simulink model "ARC_DTm"  (R2025b)
settings: Solver=FixedStepAuto  StartTime=0.0  StopTime=10080  FixedStep=1  RelTol=1e-3
PreLoadFcn:
  | %For Preload, set the working path
  | modelFolder = fileparts(which(bdroot));
  | addpath(genpath(modelFolder));
StartFcn:
  | tic
StopFcn:
  | fprintf("Sim Time: %.02f min", toc/60)
values from neighbouring files (symbols this model uses):
  batteryScenario = p.batteryScenario    [RUNSIM_ParameterSweep.m]    (also in _RUNSIM_ParameterSweep.m)
  Electricity_SalePriceModifier = 50/100    (= 0.5)    [RUNSIM_ParameterSweep.m]    (also in _RUNSIM_ParameterSweep.m)
  LUT = LUT_load.gamLUT    [RUNSIM_ParameterSweep.m]    (also in _RUNSIM_ParameterSweep.m)
  minimum_UF_system_flow = 5833    [RUNSIM_ParameterSweep.m]    (also in _RUNSIM_ParameterSweep.m)
  PROS1_recoveryrate = 61    [RUNSIM_ParameterSweep.m]    (also in _RUNSIM_ParameterSweep.m)
  PROS2_recoveryrate = 62    [RUNSIM_ParameterSweep.m]    (also in _RUNSIM_ParameterSweep.m)
  ROstabilization_time = p.ROstabilization_time    [RUNSIM_ParameterSweep.m]    (also in _RUNSIM_ParameterSweep.m)
  solarModifier = maximum_solar_generation / 300    [RUNSIM_ParameterSweep.m]    (also in _RUNSIM_ParameterSweep.m)
  TSRO_recoveryrate = 51    [RUNSIM_ParameterSweep.m]    (also in _RUNSIM_ParameterSweep.m)
  UF_RecoveryRate = 96    [RUNSIM_ParameterSweep.m]    (also in _RUNSIM_ParameterSweep.m)
undefined symbols (not defined in the file or in its folder): A_PROS1, A_PROS2, A_TSRO, B_PROS1, B_PROS2, B_TSRO, BW_Max_Time, BW_Max_Vol_gal, CEB_Max_Time, CEB_Max_Vol_gal, CIP_Max_Time, E, FF, h, L, w
libraries: simulink x40
(part 5 of 11)

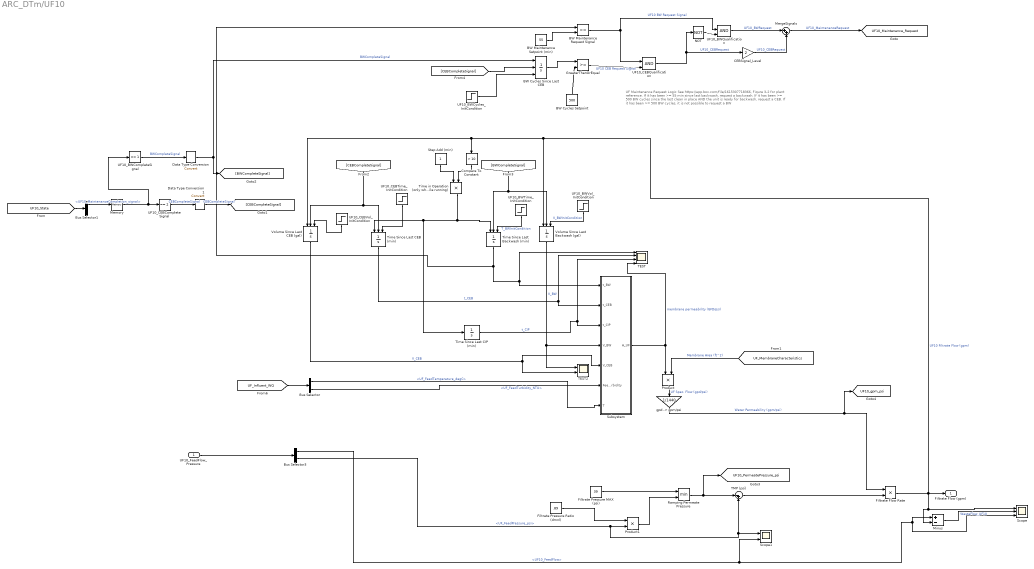
== system ARC_DTm/UF10 ==
  note: UF Maintenance Request Logic
      | See https://app.box.com/file/1615307718366, Figure 3-2 for plant reference.
      |
      | If it has been >= 55 min since last backwash, request a backwash.
      | If it has been >= 500 BW cycles since the last clean in place AND the unit is ready for backwash, request a CEB.
      | If it has been >= 500 BW cycles, it is not possible to request a BW
  UF10_FeedFlow_Pressure : Inport
  BW Cycles Setpoint : Constant  Value=500
  BW Cycles Since Last CEB : Integrator  ExternalReset=rising  InitialConditionSource=external  InitialCondition=5
  BW Maintenance Request Signal : RelationalOperator  OutDataTypeStr=boolean  RndMeth=Simplest  InputSameDT=off
  BW Maintenance Setpoint (min) : Constant  Value=55
  Bus Selector : BusSelector  OutputSignals=UF_FeedTemperature_degC,UF_FeedTurbidity_NTU
  Bus Selector1 : BusSelector  OutputSignals=UF10_MaintenanceCompletion_signal,UF10_OperationsState_signal
  Bus Selector3 : BusSelector  OutputSignals=UF10_FeedFlow,UF_FeedPressure_psi
  CEBSignal_Level : Gain  Gain=2  OutDataTypeStr=double
  Compare To Constant : simulink/Logic and Bit Operations/Compare To Constant  relop=>  const=10  OutDataTypeStr=boolean
  Data Type Conversion : DataTypeConversion  SaturateOnIntegerOverflow=off  RndMeth=Floor
  Data Type Conversion1 : DataTypeConversion  SaturateOnIntegerOverflow=off  RndMeth=Floor
  Filtrate Flow Rate : Product
  Filtrate Pressure MAX (psi) : Constant  Value=39
  Filtrate Pressure Ratio (dmnl) : Constant  Value=.89
  GreaterThanOrEqual : RelationalOperator  OutDataTypeStr=boolean  RndMeth=Simplest  InputSameDT=off
  Memory : Memory
  MergeSignals : Sum  Inputs=|++
  Minus : Sum  Inputs=+-
  NOT : Logic  Operator=NOT  IconShape=distinctive  AllPortsSameDT=off  OutDataTypeStr=boolean
  Product : Product
  Product1 : Product
  Ramping Permeate Pressure : MinMax  Inputs=2
  Scope : Scope  NumInputPorts=3
      settings: ActiveDisplayYMinimum=-126.71796384165732  ActiveDisplayYMaximum=1140.4616745749161  DataLoggingVariableName=ScopeData10
  Scope1 : Scope  NumInputPorts=2
      settings: ActiveDisplayYMinimum=-129.2228584451866  ActiveDisplayYMaximum=1163.0057260066797  DataLoggingVariableName=ScopeData11
  Step Add (min) : Constant
  Subsystem : Subsystem
  TEST : Scope  NumInputPorts=4
      settings: ActiveDisplayYMinimum=13.625  ActiveDisplayYMaximum=27.375  DataLoggingVariableName=ScopeData3
  TEST2 : Scope  NumInputPorts=2
      settings: ActiveDisplayYMinimum=-311929.86683332996  ActiveDisplayYMaximum=2.8073688014999703E+6  DataLoggingVariableName=ScopeData4
  TMP (psi) : Sum  Inputs=|-+
  Time Since Last Backwash (min) : Integrator  ExternalReset=level hold  InitialConditionSource=external  InitialCondition=26
  Time Since Last CEB (min) : Integrator  ExternalReset=level hold  InitialConditionSource=external  InitialCondition=4833
  Time Since Last CIP (min) : Integrator  InitialCondition=round(CIP_Max_Time*rand())
  Time in Operation (only while running) : Product
  UF10_BWCompleteSignal : simulink/Logic and Bit Operations/Compare To Constant  relop===  const=1  OutDataTypeStr=uint8
  UF10_BWCycles_InitCondition : Step  Before=round(500 * rand())  After=0  SampleTime=0
  UF10_BWQualification : Logic  IconShape=distinctive  AllPortsSameDT=off  OutDataTypeStr=boolean
  UF10_BWTime_InitCondition : Step  Before=round(BW_Max_Time*rand())  After=0  SampleTime=0
  UF10_BWVol_InitCondition : Step  Before=round(BW_Max_Vol_gal*rand())  After=0  SampleTime=0
  UF10_CEBCompleteSignal : simulink/Logic and Bit Operations/Compare To Constant  relop===  const=2  OutDataTypeStr=uint8
  UF10_CEBQualification : Logic  IconShape=distinctive  AllPortsSameDT=off  OutDataTypeStr=boolean
  UF10_CEBTime_InitCondition : Step  Before=round(CEB_Max_Time*rand())  After=0  SampleTime=0
  UF10_CEBVol_InitCondition : Step  Before=round(CEB_Max_Vol_gal*rand())  After=0  SampleTime=0
  Volume Since Last Backwash (gal) : Integrator  ExternalReset=level hold  InitialConditionSource=external  InitialCondition=34330
  Volume Since Last CEB (gal) : Integrator  ExternalReset=rising  InitialConditionSource=external  InitialCondition=2777254
  "gpd -> gpm/psi" : Gain  Gain=1/1440
  Filtrate Flow (gpm) : Outport
  tag scope: UF10_Maintenance_Request=global, UF10_PermeatePressure_psi=global, UF10_gpm_psi=global
  wires:
  Volume Since Last Backwash (gal)/1 -> Subsystem/4(V_BW), TEST2/1  "V_BW"
  Time Since Last Backwash (min)/1 -> BW Maintenance Request Signal/1, Subsystem/1(t_BW), TEST/1
  Product/1 -> "gpd -> gpm/psi"/1  "UF Spec. Flow (gpd/psi)"
  [UF_MembraneCharacteristics] -> Product/2  "Membrane Area (ft^2)"
  "gpd -> gpm/psi"/1 -> Filtrate Flow Rate/1, [UF10_gpm_psi]  "Water Permeability (gpm/psi)"
  Time in Operation (only while running)/1 -> Time Since Last Backwash (min)/1, Time Since Last CEB (min)/1, Time Since Last CIP (min)/1
  Filtrate Flow Rate/1 -> Scope/1, Minus/2, Volume Since Last Backwash (gal)/1, Volume Since Last CEB (gal)/1, Compare To Constant/1, Filtrate Flow (gpm)/1  "UF10 Filtrate Flow (gpm)"
  Time Since Last CEB (min)/1 -> Subsystem/2(t_CEB), TEST/2  "t_CEB"
  Volume Since Last CEB (gal)/1 -> Subsystem/5(V_CEB), TEST2/2  "V_CEB"
  Time Since Last CIP (min)/1 -> Subsystem/3(t_CIP), TEST/3  "t_CIP"
  Filtrate Pressure MAX (psi)/1 -> Ramping Permeate Pressure/1
  [UF_Influent_WQ] -> Bus Selector/1
  Bus Selector/1 -> Subsystem/7(T)  "<UF_FeedTemperature_degC>"
  UF10_FeedFlow_Pressure/1 -> Bus Selector3/1
  Filtrate Pressure Ratio (dmnl)/1 -> Product1/1
  Product1/1 -> Ramping Permeate Pressure/2
  Ramping Permeate Pressure/1 -> [UF10_PermeatePressure_psi], TMP (psi)/1
  TMP (psi)/1 -> Filtrate Flow Rate/2
  BW Maintenance Setpoint (min)/1 -> BW Maintenance Request Signal/2
  BW Cycles Since Last CEB/1 -> GreaterThanOrEqual/1
  BW Cycles Setpoint/1 -> GreaterThanOrEqual/2
  Bus Selector/2 -> Subsystem/6(Feed Turbidity)  "<UF_FeedTurbidity_NTU>"
  [UF10_State] -> Bus Selector1/1
  MergeSignals/1 -> [UF10_Maintenance_Request]  "UF10_MaintenanceRequest"
  UF10_CEBCompleteSignal/1 -> Data Type Conversion1/1  "CEBCompleteSignal"
  [CEBCompleteSignal] -> Volume Since Last CEB (gal)/2, Time Since Last CEB (min)/2
  Data Type Conversion/1 -> [BWCompleteSignal], BW Cycles Since Last CEB/1  "BWCompleteSignal"
  [BWCompleteSignal] -> Volume Since Last Backwash (gal)/2, Time Since Last Backwash (min)/2
  [CEBCompleteSignal] -> BW Cycles Since Last CEB/2
  Bus Selector1/1 -> Memory/1  "<UF10_MaintenanceCompletion_signal>"
  UF10_BWCompleteSignal/1 -> Data Type Conversion/1  "BWCompleteSignal"
  Data Type Conversion1/1 -> [CEBCompleteSignal]  "CEBCompleteSignal"
  UF10_BWCycles_InitCondition/1 -> BW Cycles Since Last CEB/3
  Subsystem/1(A_UF) -> TEST/4, Product/1  "membrane permeability (GFD/psi)"
  UF10_BWTime_InitCondition/1 -> Time Since Last Backwash (min)/3  "T_BWInitCondition"
  UF10_CEBVol_InitCondition/1 -> Volume Since Last CEB (gal)/3
  UF10_CEBTime_InitCondition/1 -> Time Since Last CEB (min)/3
  UF10_BWVol_InitCondition/1 -> Volume Since Last Backwash (gal)/3  "V_BWInitCondition"
  Step Add (min)/1 -> Time in Operation (only while running)/1
  Compare To Constant/1 -> Time in Operation (only while running)/2
  Memory/1 -> UF10_BWCompleteSignal/1, UF10_CEBCompleteSignal/1
  UF10_BWQualification/1 -> MergeSignals/1  "UF10_BWRequest"
  GreaterThanOrEqual/1 -> UF10_CEBQualification/2  "UF10 CEB Request Signal"
  UF10_CEBQualification/1 -> CEBSignal_Level/1, NOT/1  "UF10_CEBRequest"
  BW Maintenance Request Signal/1 -> UF10_BWQualification/1, UF10_CEBQualification/1  "UF10 BW Request Signal"
  NOT/1 -> UF10_BWQualification/2
  CEBSignal_Level/1 -> MergeSignals/2  "UF10_CEBRequest"
  Bus Selector3/1 -> Scope1/2, Minus/1, Scope/3  "<UF10_FeedFlow>"
  Bus Selector3/2 -> TMP (psi)/2, Scope1/1, Product1/2  "<UF_FeedPressure_psi>"
  Minus/1 -> Scope/2  "WasteFlow_UF10"

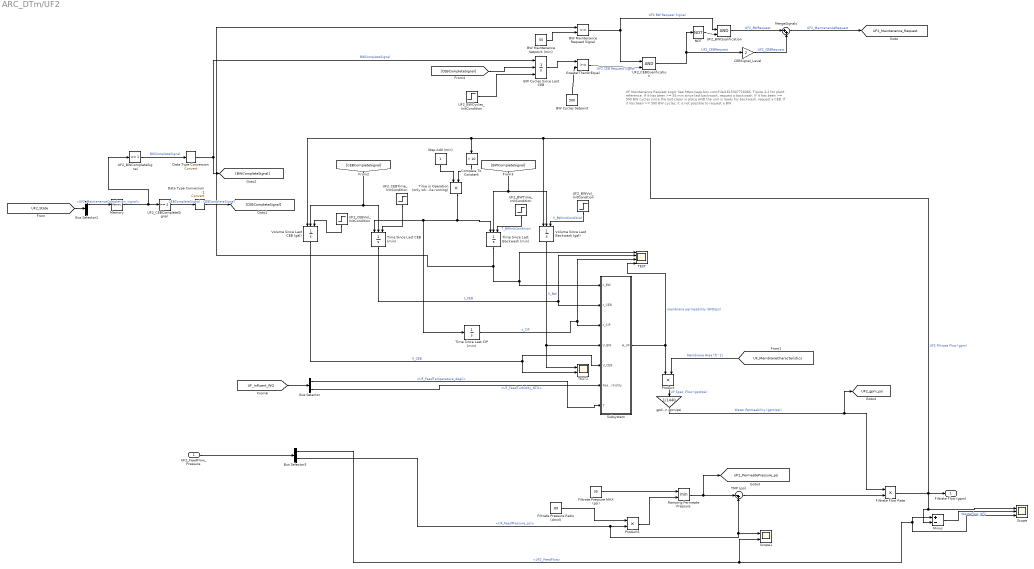
== system ARC_DTm/UF2 ==
  note: UF Maintenance Request Logic
      | See https://app.box.com/file/1615307718366, Figure 3-2 for plant reference.
      |
      | If it has been >= 55 min since last backwash, request a backwash.
      | If it has been >= 500 BW cycles since the last clean in place AND the unit is ready for backwash, request a CEB.
      | If it has been >= 500 BW cycles, it is not possible to request a BW
  UF2_FeedFlow_Pressure : Inport
  BW Cycles Setpoint : Constant  Value=500
  BW Cycles Since Last CEB : Integrator  ExternalReset=rising  InitialConditionSource=external  InitialCondition=5
  BW Maintenance Request Signal : RelationalOperator  OutDataTypeStr=boolean  RndMeth=Simplest  InputSameDT=off
  BW Maintenance Setpoint (min) : Constant  Value=55
  Bus Selector : BusSelector  OutputSignals=UF_FeedTemperature_degC,UF_FeedTurbidity_NTU
  Bus Selector1 : BusSelector  OutputSignals=UF2_MaintenanceCompletion_signal,UF2_OperationsState_signal
  Bus Selector3 : BusSelector  OutputSignals=UF2_FeedFlow,UF_FeedPressure_psi
  CEBSignal_Level : Gain  Gain=2  OutDataTypeStr=double
  Compare To Constant : simulink/Logic and Bit Operations/Compare To Constant  relop=>  const=10  OutDataTypeStr=boolean
  Data Type Conversion : DataTypeConversion  SaturateOnIntegerOverflow=off  RndMeth=Floor
  Data Type Conversion1 : DataTypeConversion  SaturateOnIntegerOverflow=off  RndMeth=Floor
  Filtrate Flow Rate : Product
  Filtrate Pressure MAX (psi) : Constant  Value=39
  Filtrate Pressure Ratio (dmnl) : Constant  Value=.89
  GreaterThanOrEqual : RelationalOperator  OutDataTypeStr=boolean  RndMeth=Simplest  InputSameDT=off
  Memory : Memory
  MergeSignals : Sum  Inputs=|++
  Minus : Sum  Inputs=+-
  NOT : Logic  Operator=NOT  IconShape=distinctive  AllPortsSameDT=off  OutDataTypeStr=boolean
  Product : Product
  Product1 : Product
  Ramping Permeate Pressure : MinMax  Inputs=2
  Scope : Scope  NumInputPorts=3
      settings: ActiveDisplayYMinimum=-126.71796384165732  ActiveDisplayYMaximum=1140.4616745749161  DataLoggingVariableName=ScopeData10
  Scope1 : Scope  NumInputPorts=2
      settings: ActiveDisplayYMinimum=-129.2228584451866  ActiveDisplayYMaximum=1163.0057260066797  DataLoggingVariableName=ScopeData11
  Step Add (min) : Constant
  Subsystem : Subsystem
  TEST : Scope  NumInputPorts=4
      settings: ActiveDisplayYMinimum=13.625  ActiveDisplayYMaximum=27.375  DataLoggingVariableName=ScopeData3
  TEST2 : Scope  NumInputPorts=2
      settings: ActiveDisplayYMinimum=-311929.86683332996  ActiveDisplayYMaximum=2.8073688014999703E+6  DataLoggingVariableName=ScopeData4
  TMP (psi) : Sum  Inputs=|-+
  Time Since Last Backwash (min) : Integrator  ExternalReset=level hold  InitialConditionSource=external  InitialCondition=26
  Time Since Last CEB (min) : Integrator  ExternalReset=level hold  InitialConditionSource=external  InitialCondition=4833
  Time Since Last CIP (min) : Integrator  InitialCondition=round(CIP_Max_Time*rand())
  Time in Operation (only while running) : Product
  UF2_BWCompleteSignal : simulink/Logic and Bit Operations/Compare To Constant  relop===  const=1  OutDataTypeStr=uint8
  UF2_BWCycles_InitCondition : Step  Before=round(500 * rand())  After=0  SampleTime=0
  UF2_BWQualification : Logic  IconShape=distinctive  AllPortsSameDT=off  OutDataTypeStr=boolean
  UF2_BWTime_InitCondition : Step  Before=round(BW_Max_Time*rand())  After=0  SampleTime=0
  UF2_BWVol_InitCondition : Step  Before=round(BW_Max_Vol_gal*rand())  After=0  SampleTime=0
  UF2_CEBCompleteSignal : simulink/Logic and Bit Operations/Compare To Constant  relop===  const=2  OutDataTypeStr=uint8
  UF2_CEBQualification : Logic  IconShape=distinctive  AllPortsSameDT=off  OutDataTypeStr=boolean
  UF2_CEBTime_InitCondition : Step  Before=round(CEB_Max_Time*rand())  After=0  SampleTime=0
  UF2_CEBVol_InitCondition : Step  Before=round(CEB_Max_Vol_gal*rand())  After=0  SampleTime=0
  Volume Since Last Backwash (gal) : Integrator  ExternalReset=level hold  InitialConditionSource=external  InitialCondition=34330
  Volume Since Last CEB (gal) : Integrator  ExternalReset=rising  InitialConditionSource=external  InitialCondition=2777254
  "gpd -> gpm/psi" : Gain  Gain=1/1440
  Filtrate Flow (gpm) : Outport
  tag scope: UF2_Maintenance_Request=global, UF2_PermeatePressure_psi=global, UF2_gpm_psi=global
  wires:
  Volume Since Last Backwash (gal)/1 -> Subsystem/4(V_BW), TEST2/1  "V_BW"
  Time Since Last Backwash (min)/1 -> BW Maintenance Request Signal/1, Subsystem/1(t_BW), TEST/1
  Product/1 -> "gpd -> gpm/psi"/1  "UF Spec. Flow (gpd/psi)"
  [UF_MembraneCharacteristics] -> Product/2  "Membrane Area (ft^2)"
  "gpd -> gpm/psi"/1 -> Filtrate Flow Rate/1, [UF2_gpm_psi]  "Water Permeability (gpm/psi)"
  Time in Operation (only while running)/1 -> Time Since Last Backwash (min)/1, Time Since Last CEB (min)/1, Time Since Last CIP (min)/1
  Filtrate Flow Rate/1 -> Scope/1, Minus/2, Volume Since Last Backwash (gal)/1, Volume Since Last CEB (gal)/1, Compare To Constant/1, Filtrate Flow (gpm)/1  "UF2 Filtrate Flow (gpm)"
  Time Since Last CEB (min)/1 -> Subsystem/2(t_CEB), TEST/2  "t_CEB"
  Volume Since Last CEB (gal)/1 -> Subsystem/5(V_CEB), TEST2/2  "V_CEB"
  Time Since Last CIP (min)/1 -> Subsystem/3(t_CIP), TEST/3  "t_CIP"
  Filtrate Pressure MAX (psi)/1 -> Ramping Permeate Pressure/1
  [UF_Influent_WQ] -> Bus Selector/1
  Bus Selector/1 -> Subsystem/7(T)  "<UF_FeedTemperature_degC>"
  UF2_FeedFlow_Pressure/1 -> Bus Selector3/1
  Filtrate Pressure Ratio (dmnl)/1 -> Product1/1
  Product1/1 -> Ramping Permeate Pressure/2
  Ramping Permeate Pressure/1 -> [UF2_PermeatePressure_psi], TMP (psi)/1
  TMP (psi)/1 -> Filtrate Flow Rate/2
  BW Maintenance Setpoint (min)/1 -> BW Maintenance Request Signal/2
  BW Cycles Since Last CEB/1 -> GreaterThanOrEqual/1
  BW Cycles Setpoint/1 -> GreaterThanOrEqual/2
  Bus Selector/2 -> Subsystem/6(Feed Turbidity)  "<UF_FeedTurbidity_NTU>"
  [UF2_State] -> Bus Selector1/1
  MergeSignals/1 -> [UF2_Maintenance_Request]  "UF2_MaintenanceRequest"
  UF2_CEBCompleteSignal/1 -> Data Type Conversion1/1  "CEBCompleteSignal"
  [CEBCompleteSignal] -> Volume Since Last CEB (gal)/2, Time Since Last CEB (min)/2
  Data Type Conversion/1 -> [BWCompleteSignal], BW Cycles Since Last CEB/1  "BWCompleteSignal"
  [BWCompleteSignal] -> Volume Since Last Backwash (gal)/2, Time Since Last Backwash (min)/2
  [CEBCompleteSignal] -> BW Cycles Since Last CEB/2
  Bus Selector1/1 -> Memory/1  "<UF2_MaintenanceCompletion_signal>"
  UF2_BWCompleteSignal/1 -> Data Type Conversion/1  "BWCompleteSignal"
  Data Type Conversion1/1 -> [CEBCompleteSignal]  "CEBCompleteSignal"
  UF2_BWCycles_InitCondition/1 -> BW Cycles Since Last CEB/3
  Subsystem/1(A_UF) -> TEST/4, Product/1  "membrane permeability (GFD/psi)"
  UF2_BWTime_InitCondition/1 -> Time Since Last Backwash (min)/3  "T_BWInitCondition"
  UF2_CEBVol_InitCondition/1 -> Volume Since Last CEB (gal)/3
  UF2_CEBTime_InitCondition/1 -> Time Since Last CEB (min)/3
  UF2_BWVol_InitCondition/1 -> Volume Since Last Backwash (gal)/3  "V_BWInitCondition"
  Step Add (min)/1 -> Time in Operation (only while running)/1
  Compare To Constant/1 -> Time in Operation (only while running)/2
  Memory/1 -> UF2_BWCompleteSignal/1, UF2_CEBCompleteSignal/1
  UF2_BWQualification/1 -> MergeSignals/1  "UF2_BWRequest"
  GreaterThanOrEqual/1 -> UF2_CEBQualification/2  "UF2 CEB Request Signal"
  UF2_CEBQualification/1 -> CEBSignal_Level/1, NOT/1  "UF2_CEBRequest"
  BW Maintenance Request Signal/1 -> UF2_BWQualification/1, UF2_CEBQualification/1  "UF2 BW Request Signal"
  NOT/1 -> UF2_BWQualification/2
  CEBSignal_Level/1 -> MergeSignals/2  "UF2_CEBRequest"
  Bus Selector3/1 -> Scope1/2, Minus/1, Scope/3  "<UF2_FeedFlow>"
  Bus Selector3/2 -> TMP (psi)/2, Scope1/1, Product1/2  "<UF_FeedPressure_psi>"
  Minus/1 -> Scope/2  "WasteFlow_UF2"

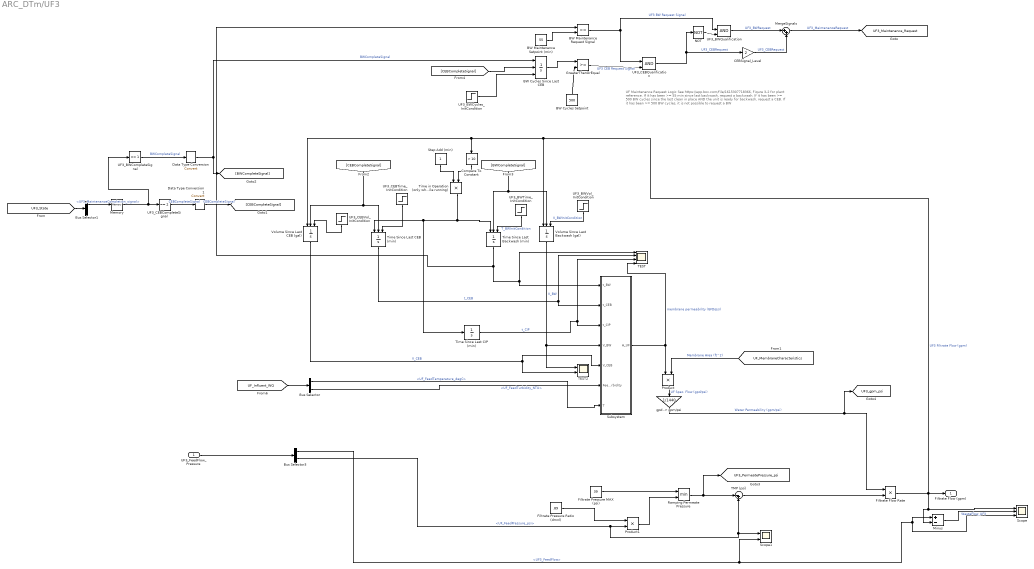
== system ARC_DTm/UF3 ==
  note: UF Maintenance Request Logic
      | See https://app.box.com/file/1615307718366, Figure 3-2 for plant reference.
      |
      | If it has been >= 55 min since last backwash, request a backwash.
      | If it has been >= 500 BW cycles since the last clean in place AND the unit is ready for backwash, request a CEB.
      | If it has been >= 500 BW cycles, it is not possible to request a BW
  UF3_FeedFlow_Pressure : Inport
  BW Cycles Setpoint : Constant  Value=500
  BW Cycles Since Last CEB : Integrator  ExternalReset=rising  InitialConditionSource=external  InitialCondition=5
  BW Maintenance Request Signal : RelationalOperator  OutDataTypeStr=boolean  RndMeth=Simplest  InputSameDT=off
  BW Maintenance Setpoint (min) : Constant  Value=55
  Bus Selector : BusSelector  OutputSignals=UF_FeedTemperature_degC,UF_FeedTurbidity_NTU
  Bus Selector1 : BusSelector  OutputSignals=UF3_MaintenanceCompletion_signal,UF3_OperationsState_signal
  Bus Selector3 : BusSelector  OutputSignals=UF3_FeedFlow,UF_FeedPressure_psi
  CEBSignal_Level : Gain  Gain=2  OutDataTypeStr=double
  Compare To Constant : simulink/Logic and Bit Operations/Compare To Constant  relop=>  const=10  OutDataTypeStr=boolean
  Data Type Conversion : DataTypeConversion  SaturateOnIntegerOverflow=off  RndMeth=Floor
  Data Type Conversion1 : DataTypeConversion  SaturateOnIntegerOverflow=off  RndMeth=Floor
  Filtrate Flow Rate : Product
  Filtrate Pressure MAX (psi) : Constant  Value=39
  Filtrate Pressure Ratio (dmnl) : Constant  Value=.89
  GreaterThanOrEqual : RelationalOperator  OutDataTypeStr=boolean  RndMeth=Simplest  InputSameDT=off
  Memory : Memory
  MergeSignals : Sum  Inputs=|++
  Minus : Sum  Inputs=+-
  NOT : Logic  Operator=NOT  IconShape=distinctive  AllPortsSameDT=off  OutDataTypeStr=boolean
  Product : Product
  Product1 : Product
  Ramping Permeate Pressure : MinMax  Inputs=2
  Scope : Scope  NumInputPorts=3
      settings: ActiveDisplayYMinimum=-126.71796384165732  ActiveDisplayYMaximum=1140.4616745749161  DataLoggingVariableName=ScopeData10
  Scope1 : Scope  NumInputPorts=2
      settings: ActiveDisplayYMinimum=-129.2228584451866  ActiveDisplayYMaximum=1163.0057260066797  DataLoggingVariableName=ScopeData11
  Step Add (min) : Constant
  Subsystem : Subsystem
  TEST : Scope  NumInputPorts=4
      settings: ActiveDisplayYMinimum=13.625  ActiveDisplayYMaximum=27.375  DataLoggingVariableName=ScopeData3
  TEST2 : Scope  NumInputPorts=2
      settings: ActiveDisplayYMinimum=-311929.86683332996  ActiveDisplayYMaximum=2.8073688014999703E+6  DataLoggingVariableName=ScopeData4
  TMP (psi) : Sum  Inputs=|-+
  Time Since Last Backwash (min) : Integrator  ExternalReset=level hold  InitialConditionSource=external  InitialCondition=26
  Time Since Last CEB (min) : Integrator  ExternalReset=level hold  InitialConditionSource=external  InitialCondition=4833
  Time Since Last CIP (min) : Integrator  InitialCondition=round(CIP_Max_Time*rand())
  Time in Operation (only while running) : Product
  UF3_BWCompleteSignal : simulink/Logic and Bit Operations/Compare To Constant  relop===  const=1  OutDataTypeStr=uint8
  UF3_BWCycles_InitCondition : Step  Before=round(500 * rand())  After=0  SampleTime=0
  UF3_BWQualification : Logic  IconShape=distinctive  AllPortsSameDT=off  OutDataTypeStr=boolean
  UF3_BWTime_InitCondition : Step  Before=round(BW_Max_Time*rand())  After=0  SampleTime=0
  UF3_BWVol_InitCondition : Step  Before=round(BW_Max_Vol_gal*rand())  After=0  SampleTime=0
  UF3_CEBCompleteSignal : simulink/Logic and Bit Operations/Compare To Constant  relop===  const=2  OutDataTypeStr=uint8
  UF3_CEBQualification : Logic  IconShape=distinctive  AllPortsSameDT=off  OutDataTypeStr=boolean
  UF3_CEBTime_InitCondition : Step  Before=round(CEB_Max_Time*rand())  After=0  SampleTime=0
  UF3_CEBVol_InitCondition : Step  Before=round(CEB_Max_Vol_gal*rand())  After=0  SampleTime=0
  Volume Since Last Backwash (gal) : Integrator  ExternalReset=level hold  InitialConditionSource=external  InitialCondition=34330
  Volume Since Last CEB (gal) : Integrator  ExternalReset=rising  InitialConditionSource=external  InitialCondition=2777254
  "gpd -> gpm/psi" : Gain  Gain=1/1440
  Filtrate Flow (gpm) : Outport
  tag scope: UF3_Maintenance_Request=global, UF3_PermeatePressure_psi=global, UF3_gpm_psi=global
  wires:
  Volume Since Last Backwash (gal)/1 -> Subsystem/4(V_BW), TEST2/1  "V_BW"
  Time Since Last Backwash (min)/1 -> BW Maintenance Request Signal/1, Subsystem/1(t_BW), TEST/1
  Product/1 -> "gpd -> gpm/psi"/1  "UF Spec. Flow (gpd/psi)"
  [UF_MembraneCharacteristics] -> Product/2  "Membrane Area (ft^2)"
  "gpd -> gpm/psi"/1 -> Filtrate Flow Rate/1, [UF3_gpm_psi]  "Water Permeability (gpm/psi)"
  Time in Operation (only while running)/1 -> Time Since Last Backwash (min)/1, Time Since Last CEB (min)/1, Time Since Last CIP (min)/1
  Filtrate Flow Rate/1 -> Scope/1, Minus/2, Volume Since Last Backwash (gal)/1, Volume Since Last CEB (gal)/1, Compare To Constant/1, Filtrate Flow (gpm)/1  "UF3 Filtrate Flow (gpm)"
  Time Since Last CEB (min)/1 -> Subsystem/2(t_CEB), TEST/2  "t_CEB"
  Volume Since Last CEB (gal)/1 -> Subsystem/5(V_CEB), TEST2/2  "V_CEB"
  Time Since Last CIP (min)/1 -> Subsystem/3(t_CIP), TEST/3  "t_CIP"
  Filtrate Pressure MAX (psi)/1 -> Ramping Permeate Pressure/1
  [UF_Influent_WQ] -> Bus Selector/1
  Bus Selector/1 -> Subsystem/7(T)  "<UF_FeedTemperature_degC>"
  UF3_FeedFlow_Pressure/1 -> Bus Selector3/1
  Filtrate Pressure Ratio (dmnl)/1 -> Product1/1
  Product1/1 -> Ramping Permeate Pressure/2
  Ramping Permeate Pressure/1 -> [UF3_PermeatePressure_psi], TMP (psi)/1
  TMP (psi)/1 -> Filtrate Flow Rate/2
  BW Maintenance Setpoint (min)/1 -> BW Maintenance Request Signal/2
  BW Cycles Since Last CEB/1 -> GreaterThanOrEqual/1
  BW Cycles Setpoint/1 -> GreaterThanOrEqual/2
  Bus Selector/2 -> Subsystem/6(Feed Turbidity)  "<UF_FeedTurbidity_NTU>"
  [UF3_State] -> Bus Selector1/1
  MergeSignals/1 -> [UF3_Maintenance_Request]  "UF3_MaintenanceRequest"
  UF3_CEBCompleteSignal/1 -> Data Type Conversion1/1  "CEBCompleteSignal"
  [CEBCompleteSignal] -> Volume Since Last CEB (gal)/2, Time Since Last CEB (min)/2
  Data Type Conversion/1 -> [BWCompleteSignal], BW Cycles Since Last CEB/1  "BWCompleteSignal"
  [BWCompleteSignal] -> Volume Since Last Backwash (gal)/2, Time Since Last Backwash (min)/2
  [CEBCompleteSignal] -> BW Cycles Since Last CEB/2
  Bus Selector1/1 -> Memory/1  "<UF3_MaintenanceCompletion_signal>"
  UF3_BWCompleteSignal/1 -> Data Type Conversion/1  "BWCompleteSignal"
  Data Type Conversion1/1 -> [CEBCompleteSignal]  "CEBCompleteSignal"
  UF3_BWCycles_InitCondition/1 -> BW Cycles Since Last CEB/3
  Subsystem/1(A_UF) -> TEST/4, Product/1  "membrane permeability (GFD/psi)"
  UF3_BWTime_InitCondition/1 -> Time Since Last Backwash (min)/3  "T_BWInitCondition"
  UF3_CEBVol_InitCondition/1 -> Volume Since Last CEB (gal)/3
  UF3_CEBTime_InitCondition/1 -> Time Since Last CEB (min)/3
  UF3_BWVol_InitCondition/1 -> Volume Since Last Backwash (gal)/3  "V_BWInitCondition"
  Step Add (min)/1 -> Time in Operation (only while running)/1
  Compare To Constant/1 -> Time in Operation (only while running)/2
  Memory/1 -> UF3_BWCompleteSignal/1, UF3_CEBCompleteSignal/1
  UF3_BWQualification/1 -> MergeSignals/1  "UF3_BWRequest"
  GreaterThanOrEqual/1 -> UF3_CEBQualification/2  "UF3 CEB Request Signal"
  UF3_CEBQualification/1 -> CEBSignal_Level/1, NOT/1  "UF3_CEBRequest"
  BW Maintenance Request Signal/1 -> UF3_BWQualification/1, UF3_CEBQualification/1  "UF3 BW Request Signal"
  NOT/1 -> UF3_BWQualification/2
  CEBSignal_Level/1 -> MergeSignals/2  "UF3_CEBRequest"
  Bus Selector3/1 -> Scope1/2, Minus/1, Scope/3  "<UF3_FeedFlow>"
  Bus Selector3/2 -> TMP (psi)/2, Scope1/1, Product1/2  "<UF_FeedPressure_psi>"
  Minus/1 -> Scope/2  "WasteFlow_UF3"

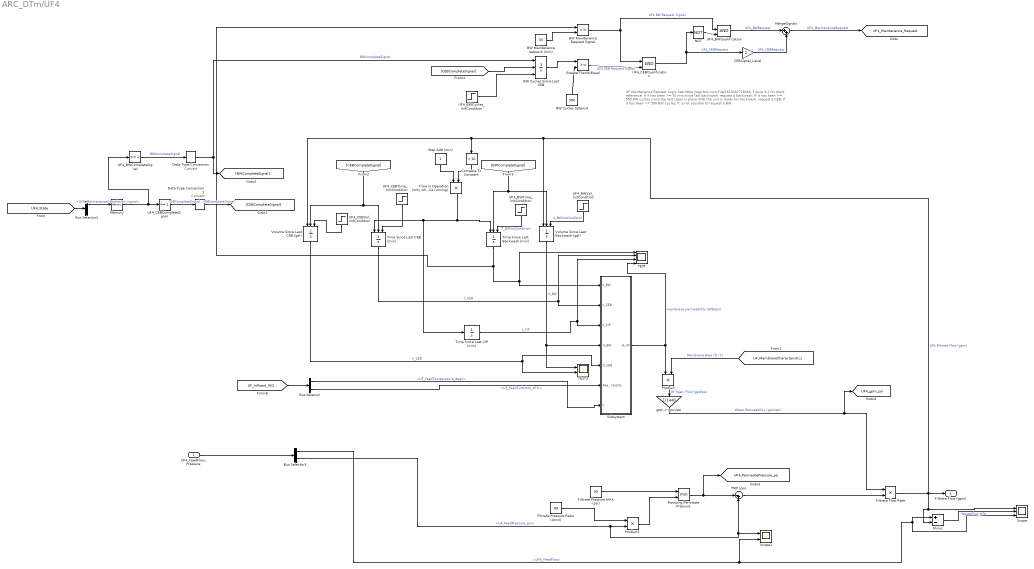
== system ARC_DTm/UF4 ==
  note: UF Maintenance Request Logic
      | See https://app.box.com/file/1615307718366, Figure 3-2 for plant reference.
      |
      | If it has been >= 55 min since last backwash, request a backwash.
      | If it has been >= 500 BW cycles since the last clean in place AND the unit is ready for backwash, request a CEB.
      | If it has been >= 500 BW cycles, it is not possible to request a BW
  UF4_FeedFlow_Pressure : Inport
  BW Cycles Setpoint : Constant  Value=500
  BW Cycles Since Last CEB : Integrator  ExternalReset=rising  InitialConditionSource=external  InitialCondition=5
  BW Maintenance Request Signal : RelationalOperator  OutDataTypeStr=boolean  RndMeth=Simplest  InputSameDT=off
  BW Maintenance Setpoint (min) : Constant  Value=55
  Bus Selector : BusSelector  OutputSignals=UF_FeedTemperature_degC,UF_FeedTurbidity_NTU
  Bus Selector1 : BusSelector  OutputSignals=UF4_MaintenanceCompletion_signal,UF4_OperationsState_signal
  Bus Selector3 : BusSelector  OutputSignals=UF4_FeedFlow,UF_FeedPressure_psi
  CEBSignal_Level : Gain  Gain=2  OutDataTypeStr=double
  Compare To Constant : simulink/Logic and Bit Operations/Compare To Constant  relop=>  const=10  OutDataTypeStr=boolean
  Data Type Conversion : DataTypeConversion  SaturateOnIntegerOverflow=off  RndMeth=Floor
  Data Type Conversion1 : DataTypeConversion  SaturateOnIntegerOverflow=off  RndMeth=Floor
  Filtrate Flow Rate : Product
  Filtrate Pressure MAX (psi) : Constant  Value=39
  Filtrate Pressure Ratio (dmnl) : Constant  Value=.89
  GreaterThanOrEqual : RelationalOperator  OutDataTypeStr=boolean  RndMeth=Simplest  InputSameDT=off
  Memory : Memory
  MergeSignals : Sum  Inputs=|++
  Minus : Sum  Inputs=+-
  NOT : Logic  Operator=NOT  IconShape=distinctive  AllPortsSameDT=off  OutDataTypeStr=boolean
  Product : Product
  Product1 : Product
  Ramping Permeate Pressure : MinMax  Inputs=2
  Scope : Scope  NumInputPorts=3
      settings: ActiveDisplayYMinimum=-126.71796384165732  ActiveDisplayYMaximum=1140.4616745749161  DataLoggingVariableName=ScopeData10
  Scope1 : Scope  NumInputPorts=2
      settings: ActiveDisplayYMinimum=-129.2228584451866  ActiveDisplayYMaximum=1163.0057260066797  DataLoggingVariableName=ScopeData11
  Step Add (min) : Constant
  Subsystem : Subsystem
  TEST : Scope  NumInputPorts=4
      settings: ActiveDisplayYMinimum=13.625  ActiveDisplayYMaximum=27.375  DataLoggingVariableName=ScopeData3
  TEST2 : Scope  NumInputPorts=2
      settings: ActiveDisplayYMinimum=-311929.86683332996  ActiveDisplayYMaximum=2.8073688014999703E+6  DataLoggingVariableName=ScopeData4
  TMP (psi) : Sum  Inputs=|-+
  Time Since Last Backwash (min) : Integrator  ExternalReset=level hold  InitialConditionSource=external  InitialCondition=26
  Time Since Last CEB (min) : Integrator  ExternalReset=level hold  InitialConditionSource=external  InitialCondition=4833
  Time Since Last CIP (min) : Integrator  InitialCondition=round(CIP_Max_Time*rand())
  Time in Operation (only while running) : Product
  UF4_BWCompleteSignal : simulink/Logic and Bit Operations/Compare To Constant  relop===  const=1  OutDataTypeStr=uint8
  UF4_BWCycles_InitCondition : Step  Before=round(500 * rand())  After=0  SampleTime=0
  UF4_BWQualification : Logic  IconShape=distinctive  AllPortsSameDT=off  OutDataTypeStr=boolean
  UF4_BWTime_InitCondition : Step  Before=round(BW_Max_Time*rand())  After=0  SampleTime=0
  UF4_BWVol_InitCondition : Step  Before=round(BW_Max_Vol_gal*rand())  After=0  SampleTime=0
  UF4_CEBCompleteSignal : simulink/Logic and Bit Operations/Compare To Constant  relop===  const=2  OutDataTypeStr=uint8
  UF4_CEBQualification : Logic  IconShape=distinctive  AllPortsSameDT=off  OutDataTypeStr=boolean
  UF4_CEBTime_InitCondition : Step  Before=round(CEB_Max_Time*rand())  After=0  SampleTime=0
  UF4_CEBVol_InitCondition : Step  Before=round(CEB_Max_Vol_gal*rand())  After=0  SampleTime=0
  Volume Since Last Backwash (gal) : Integrator  ExternalReset=level hold  InitialConditionSource=external  InitialCondition=34330
  Volume Since Last CEB (gal) : Integrator  ExternalReset=rising  InitialConditionSource=external  InitialCondition=2777254
  "gpd -> gpm/psi" : Gain  Gain=1/1440
  Filtrate Flow (gpm) : Outport
  tag scope: UF4_Maintenance_Request=global, UF4_PermeatePressure_psi=global, UF4_gpm_psi=global
  wires:
  Volume Since Last Backwash (gal)/1 -> Subsystem/4(V_BW), TEST2/1  "V_BW"
  Time Since Last Backwash (min)/1 -> BW Maintenance Request Signal/1, Subsystem/1(t_BW), TEST/1
  Product/1 -> "gpd -> gpm/psi"/1  "UF Spec. Flow (gpd/psi)"
  [UF_MembraneCharacteristics] -> Product/2  "Membrane Area (ft^2)"
  "gpd -> gpm/psi"/1 -> Filtrate Flow Rate/1, [UF4_gpm_psi]  "Water Permeability (gpm/psi)"
  Time in Operation (only while running)/1 -> Time Since Last Backwash (min)/1, Time Since Last CEB (min)/1, Time Since Last CIP (min)/1
  Filtrate Flow Rate/1 -> Scope/1, Minus/2, Volume Since Last Backwash (gal)/1, Volume Since Last CEB (gal)/1, Compare To Constant/1, Filtrate Flow (gpm)/1  "UF4 Filtrate Flow (gpm)"
  Time Since Last CEB (min)/1 -> Subsystem/2(t_CEB), TEST/2  "t_CEB"
  Volume Since Last CEB (gal)/1 -> Subsystem/5(V_CEB), TEST2/2  "V_CEB"
  Time Since Last CIP (min)/1 -> Subsystem/3(t_CIP), TEST/3  "t_CIP"
  Filtrate Pressure MAX (psi)/1 -> Ramping Permeate Pressure/1
  [UF_Influent_WQ] -> Bus Selector/1
  Bus Selector/1 -> Subsystem/7(T)  "<UF_FeedTemperature_degC>"
  UF4_FeedFlow_Pressure/1 -> Bus Selector3/1
  Filtrate Pressure Ratio (dmnl)/1 -> Product1/1
  Product1/1 -> Ramping Permeate Pressure/2
  Ramping Permeate Pressure/1 -> [UF4_PermeatePressure_psi], TMP (psi)/1
  TMP (psi)/1 -> Filtrate Flow Rate/2
  BW Maintenance Setpoint (min)/1 -> BW Maintenance Request Signal/2
  BW Cycles Since Last CEB/1 -> GreaterThanOrEqual/1
  BW Cycles Setpoint/1 -> GreaterThanOrEqual/2
  Bus Selector/2 -> Subsystem/6(Feed Turbidity)  "<UF_FeedTurbidity_NTU>"
  [UF4_State] -> Bus Selector1/1
  MergeSignals/1 -> [UF4_Maintenance_Request]  "UF4_MaintenanceRequest"
  UF4_CEBCompleteSignal/1 -> Data Type Conversion1/1  "CEBCompleteSignal"
  [CEBCompleteSignal] -> Volume Since Last CEB (gal)/2, Time Since Last CEB (min)/2
  Data Type Conversion/1 -> [BWCompleteSignal], BW Cycles Since Last CEB/1  "BWCompleteSignal"
  [BWCompleteSignal] -> Volume Since Last Backwash (gal)/2, Time Since Last Backwash (min)/2
  [CEBCompleteSignal] -> BW Cycles Since Last CEB/2
  Bus Selector1/1 -> Memory/1  "<UF4_MaintenanceCompletion_signal>"
  UF4_BWCompleteSignal/1 -> Data Type Conversion/1  "BWCompleteSignal"
  Data Type Conversion1/1 -> [CEBCompleteSignal]  "CEBCompleteSignal"
  UF4_BWCycles_InitCondition/1 -> BW Cycles Since Last CEB/3
  Subsystem/1(A_UF) -> TEST/4, Product/1  "membrane permeability (GFD/psi)"
  UF4_BWTime_InitCondition/1 -> Time Since Last Backwash (min)/3  "T_BWInitCondition"
  UF4_CEBVol_InitCondition/1 -> Volume Since Last CEB (gal)/3
  UF4_CEBTime_InitCondition/1 -> Time Since Last CEB (min)/3
  UF4_BWVol_InitCondition/1 -> Volume Since Last Backwash (gal)/3  "V_BWInitCondition"
  Step Add (min)/1 -> Time in Operation (only while running)/1
  Compare To Constant/1 -> Time in Operation (only while running)/2
  Memory/1 -> UF4_BWCompleteSignal/1, UF4_CEBCompleteSignal/1
  UF4_BWQualification/1 -> MergeSignals/1  "UF4_BWRequest"
  GreaterThanOrEqual/1 -> UF4_CEBQualification/2  "UF4 CEB Request Signal"
  UF4_CEBQualification/1 -> CEBSignal_Level/1, NOT/1  "UF4_CEBRequest"
  BW Maintenance Request Signal/1 -> UF4_BWQualification/1, UF4_CEBQualification/1  "UF4 BW Request Signal"
  NOT/1 -> UF4_BWQualification/2
  CEBSignal_Level/1 -> MergeSignals/2  "UF4_CEBRequest"
  Bus Selector3/1 -> Scope1/2, Minus/1, Scope/3  "<UF4_FeedFlow>"
  Bus Selector3/2 -> TMP (psi)/2, Scope1/1, Product1/2  "<UF_FeedPressure_psi>"
  Minus/1 -> Scope/2  "WasteFlow_UF4"

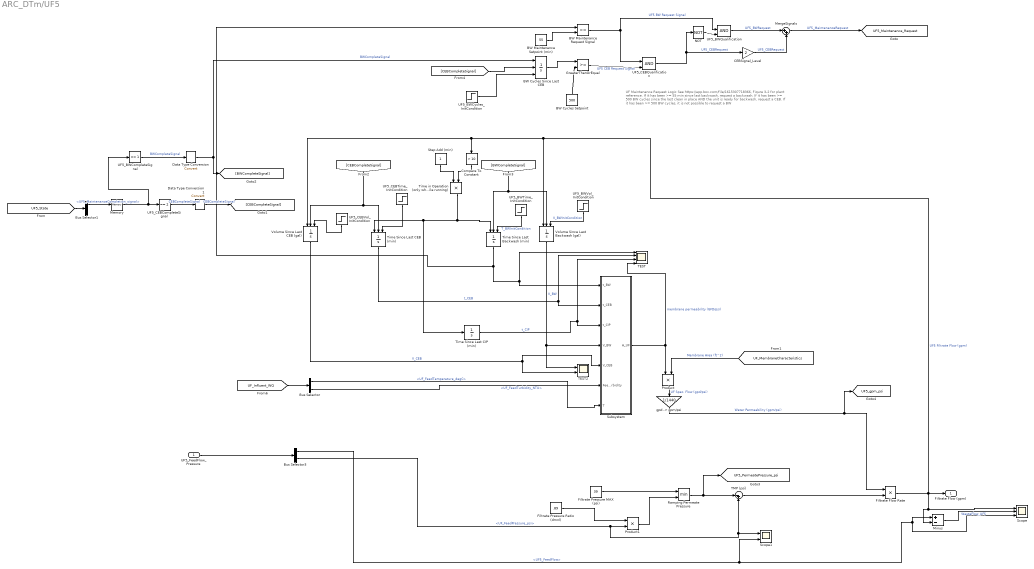
== system ARC_DTm/UF5 ==
  note: UF Maintenance Request Logic
      | See https://app.box.com/file/1615307718366, Figure 3-2 for plant reference.
      |
      | If it has been >= 55 min since last backwash, request a backwash.
      | If it has been >= 500 BW cycles since the last clean in place AND the unit is ready for backwash, request a CEB.
      | If it has been >= 500 BW cycles, it is not possible to request a BW
  UF5_FeedFlow_Pressure : Inport
  BW Cycles Setpoint : Constant  Value=500
  BW Cycles Since Last CEB : Integrator  ExternalReset=rising  InitialConditionSource=external  InitialCondition=5
  BW Maintenance Request Signal : RelationalOperator  OutDataTypeStr=boolean  RndMeth=Simplest  InputSameDT=off
  BW Maintenance Setpoint (min) : Constant  Value=55
  Bus Selector : BusSelector  OutputSignals=UF_FeedTemperature_degC,UF_FeedTurbidity_NTU
  Bus Selector1 : BusSelector  OutputSignals=UF5_MaintenanceCompletion_signal,UF5_OperationsState_signal
  Bus Selector3 : BusSelector  OutputSignals=UF5_FeedFlow,UF_FeedPressure_psi
  CEBSignal_Level : Gain  Gain=2  OutDataTypeStr=double
  Compare To Constant : simulink/Logic and Bit Operations/Compare To Constant  relop=>  const=10  OutDataTypeStr=boolean
  Data Type Conversion : DataTypeConversion  SaturateOnIntegerOverflow=off  RndMeth=Floor
  Data Type Conversion1 : DataTypeConversion  SaturateOnIntegerOverflow=off  RndMeth=Floor
  Filtrate Flow Rate : Product
  Filtrate Pressure MAX (psi) : Constant  Value=39
  Filtrate Pressure Ratio (dmnl) : Constant  Value=.89
  GreaterThanOrEqual : RelationalOperator  OutDataTypeStr=boolean  RndMeth=Simplest  InputSameDT=off
  Memory : Memory
  MergeSignals : Sum  Inputs=|++
  Minus : Sum  Inputs=+-
  NOT : Logic  Operator=NOT  IconShape=distinctive  AllPortsSameDT=off  OutDataTypeStr=boolean
  Product : Product
  Product1 : Product
  Ramping Permeate Pressure : MinMax  Inputs=2
  Scope : Scope  NumInputPorts=3
      settings: ActiveDisplayYMinimum=-126.71796384165732  ActiveDisplayYMaximum=1140.4616745749161  DataLoggingVariableName=ScopeData10
  Scope1 : Scope  NumInputPorts=2
      settings: ActiveDisplayYMinimum=-129.2228584451866  ActiveDisplayYMaximum=1163.0057260066797  DataLoggingVariableName=ScopeData11
  Step Add (min) : Constant
  Subsystem : Subsystem
  TEST : Scope  NumInputPorts=4
      settings: ActiveDisplayYMinimum=13.625  ActiveDisplayYMaximum=27.375  DataLoggingVariableName=ScopeData3
  TEST2 : Scope  NumInputPorts=2
      settings: ActiveDisplayYMinimum=-311929.86683332996  ActiveDisplayYMaximum=2.8073688014999703E+6  DataLoggingVariableName=ScopeData4
  TMP (psi) : Sum  Inputs=|-+
  Time Since Last Backwash (min) : Integrator  ExternalReset=level hold  InitialConditionSource=external  InitialCondition=26
  Time Since Last CEB (min) : Integrator  ExternalReset=level hold  InitialConditionSource=external  InitialCondition=4833
  Time Since Last CIP (min) : Integrator  InitialCondition=round(CIP_Max_Time*rand())
  Time in Operation (only while running) : Product
  UF5_BWCompleteSignal : simulink/Logic and Bit Operations/Compare To Constant  relop===  const=1  OutDataTypeStr=uint8
  UF5_BWCycles_InitCondition : Step  Before=round(500 * rand())  After=0  SampleTime=0
  UF5_BWQualification : Logic  IconShape=distinctive  AllPortsSameDT=off  OutDataTypeStr=boolean
  UF5_BWTime_InitCondition : Step  Before=round(BW_Max_Time*rand())  After=0  SampleTime=0
  UF5_BWVol_InitCondition : Step  Before=round(BW_Max_Vol_gal*rand())  After=0  SampleTime=0
  UF5_CEBCompleteSignal : simulink/Logic and Bit Operations/Compare To Constant  relop===  const=2  OutDataTypeStr=uint8
  UF5_CEBQualification : Logic  IconShape=distinctive  AllPortsSameDT=off  OutDataTypeStr=boolean
  UF5_CEBTime_InitCondition : Step  Before=round(CEB_Max_Time*rand())  After=0  SampleTime=0
  UF5_CEBVol_InitCondition : Step  Before=round(CEB_Max_Vol_gal*rand())  After=0  SampleTime=0
  Volume Since Last Backwash (gal) : Integrator  ExternalReset=level hold  InitialConditionSource=external  InitialCondition=34330
  Volume Since Last CEB (gal) : Integrator  ExternalReset=rising  InitialConditionSource=external  InitialCondition=2777254
  "gpd -> gpm/psi" : Gain  Gain=1/1440
  Filtrate Flow (gpm) : Outport
  tag scope: UF5_Maintenance_Request=global, UF5_PermeatePressure_psi=global, UF5_gpm_psi=global
  wires:
  Volume Since Last Backwash (gal)/1 -> Subsystem/4(V_BW), TEST2/1  "V_BW"
  Time Since Last Backwash (min)/1 -> BW Maintenance Request Signal/1, Subsystem/1(t_BW), TEST/1
  Product/1 -> "gpd -> gpm/psi"/1  "UF Spec. Flow (gpd/psi)"
  [UF_MembraneCharacteristics] -> Product/2  "Membrane Area (ft^2)"
  "gpd -> gpm/psi"/1 -> Filtrate Flow Rate/1, [UF5_gpm_psi]  "Water Permeability (gpm/psi)"
  Time in Operation (only while running)/1 -> Time Since Last Backwash (min)/1, Time Since Last CEB (min)/1, Time Since Last CIP (min)/1
  Filtrate Flow Rate/1 -> Scope/1, Minus/2, Volume Since Last Backwash (gal)/1, Volume Since Last CEB (gal)/1, Compare To Constant/1, Filtrate Flow (gpm)/1  "UF5 Filtrate Flow (gpm)"
  Time Since Last CEB (min)/1 -> Subsystem/2(t_CEB), TEST/2  "t_CEB"
  Volume Since Last CEB (gal)/1 -> Subsystem/5(V_CEB), TEST2/2  "V_CEB"
  Time Since Last CIP (min)/1 -> Subsystem/3(t_CIP), TEST/3  "t_CIP"
  Filtrate Pressure MAX (psi)/1 -> Ramping Permeate Pressure/1
  [UF_Influent_WQ] -> Bus Selector/1
  Bus Selector/1 -> Subsystem/7(T)  "<UF_FeedTemperature_degC>"
  UF5_FeedFlow_Pressure/1 -> Bus Selector3/1
  Filtrate Pressure Ratio (dmnl)/1 -> Product1/1
  Product1/1 -> Ramping Permeate Pressure/2
  Ramping Permeate Pressure/1 -> [UF5_PermeatePressure_psi], TMP (psi)/1
  TMP (psi)/1 -> Filtrate Flow Rate/2
  BW Maintenance Setpoint (min)/1 -> BW Maintenance Request Signal/2
  BW Cycles Since Last CEB/1 -> GreaterThanOrEqual/1
  BW Cycles Setpoint/1 -> GreaterThanOrEqual/2
  Bus Selector/2 -> Subsystem/6(Feed Turbidity)  "<UF_FeedTurbidity_NTU>"
  [UF5_State] -> Bus Selector1/1
  MergeSignals/1 -> [UF5_Maintenance_Request]  "UF5_MaintenanceRequest"
  UF5_CEBCompleteSignal/1 -> Data Type Conversion1/1  "CEBCompleteSignal"
  [CEBCompleteSignal] -> Volume Since Last CEB (gal)/2, Time Since Last CEB (min)/2
  Data Type Conversion/1 -> [BWCompleteSignal], BW Cycles Since Last CEB/1  "BWCompleteSignal"
  [BWCompleteSignal] -> Volume Since Last Backwash (gal)/2, Time Since Last Backwash (min)/2
  [CEBCompleteSignal] -> BW Cycles Since Last CEB/2
  Bus Selector1/1 -> Memory/1  "<UF5_MaintenanceCompletion_signal>"
  UF5_BWCompleteSignal/1 -> Data Type Conversion/1  "BWCompleteSignal"
  Data Type Conversion1/1 -> [CEBCompleteSignal]  "CEBCompleteSignal"
  UF5_BWCycles_InitCondition/1 -> BW Cycles Since Last CEB/3
  Subsystem/1(A_UF) -> TEST/4, Product/1  "membrane permeability (GFD/psi)"
  UF5_BWTime_InitCondition/1 -> Time Since Last Backwash (min)/3  "T_BWInitCondition"
  UF5_CEBVol_InitCondition/1 -> Volume Since Last CEB (gal)/3
  UF5_CEBTime_InitCondition/1 -> Time Since Last CEB (min)/3
  UF5_BWVol_InitCondition/1 -> Volume Since Last Backwash (gal)/3  "V_BWInitCondition"
  Step Add (min)/1 -> Time in Operation (only while running)/1
  Compare To Constant/1 -> Time in Operation (only while running)/2
  Memory/1 -> UF5_BWCompleteSignal/1, UF5_CEBCompleteSignal/1
  UF5_BWQualification/1 -> MergeSignals/1  "UF5_BWRequest"
  GreaterThanOrEqual/1 -> UF5_CEBQualification/2  "UF5 CEB Request Signal"
  UF5_CEBQualification/1 -> CEBSignal_Level/1, NOT/1  "UF5_CEBRequest"
  BW Maintenance Request Signal/1 -> UF5_BWQualification/1, UF5_CEBQualification/1  "UF5 BW Request Signal"
  NOT/1 -> UF5_BWQualification/2
  CEBSignal_Level/1 -> MergeSignals/2  "UF5_CEBRequest"
  Bus Selector3/1 -> Scope1/2, Minus/1, Scope/3  "<UF5_FeedFlow>"
  Bus Selector3/2 -> TMP (psi)/2, Scope1/1, Product1/2  "<UF_FeedPressure_psi>"
  Minus/1 -> Scope/2  "WasteFlow_UF5"

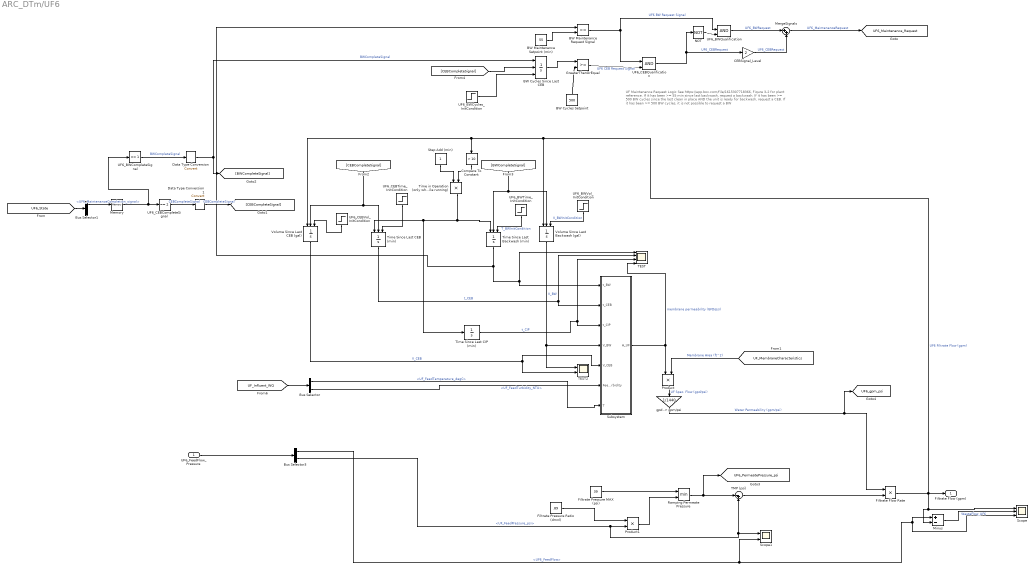
== system ARC_DTm/UF6 ==
  note: UF Maintenance Request Logic
      | See https://app.box.com/file/1615307718366, Figure 3-2 for plant reference.
      |
      | If it has been >= 55 min since last backwash, request a backwash.
      | If it has been >= 500 BW cycles since the last clean in place AND the unit is ready for backwash, request a CEB.
      | If it has been >= 500 BW cycles, it is not possible to request a BW
  UF6_FeedFlow_Pressure : Inport
  BW Cycles Setpoint : Constant  Value=500
  BW Cycles Since Last CEB : Integrator  ExternalReset=rising  InitialConditionSource=external  InitialCondition=5
  BW Maintenance Request Signal : RelationalOperator  OutDataTypeStr=boolean  RndMeth=Simplest  InputSameDT=off
  BW Maintenance Setpoint (min) : Constant  Value=55
  Bus Selector : BusSelector  OutputSignals=UF_FeedTemperature_degC,UF_FeedTurbidity_NTU
  Bus Selector1 : BusSelector  OutputSignals=UF6_MaintenanceCompletion_signal,UF6_OperationsState_signal
  Bus Selector3 : BusSelector  OutputSignals=UF6_FeedFlow,UF_FeedPressure_psi
  CEBSignal_Level : Gain  Gain=2  OutDataTypeStr=double
  Compare To Constant : simulink/Logic and Bit Operations/Compare To Constant  relop=>  const=10  OutDataTypeStr=boolean
  Data Type Conversion : DataTypeConversion  SaturateOnIntegerOverflow=off  RndMeth=Floor
  Data Type Conversion1 : DataTypeConversion  SaturateOnIntegerOverflow=off  RndMeth=Floor
  Filtrate Flow Rate : Product
  Filtrate Pressure MAX (psi) : Constant  Value=39
  Filtrate Pressure Ratio (dmnl) : Constant  Value=.89
  GreaterThanOrEqual : RelationalOperator  OutDataTypeStr=boolean  RndMeth=Simplest  InputSameDT=off
  Memory : Memory
  MergeSignals : Sum  Inputs=|++
  Minus : Sum  Inputs=+-
  NOT : Logic  Operator=NOT  IconShape=distinctive  AllPortsSameDT=off  OutDataTypeStr=boolean
  Product : Product
  Product1 : Product
  Ramping Permeate Pressure : MinMax  Inputs=2
  Scope : Scope  NumInputPorts=3
      settings: ActiveDisplayYMinimum=-126.71796384165732  ActiveDisplayYMaximum=1140.4616745749161  DataLoggingVariableName=ScopeData10
  Scope1 : Scope  NumInputPorts=2
      settings: ActiveDisplayYMinimum=-129.2228584451866  ActiveDisplayYMaximum=1163.0057260066797  DataLoggingVariableName=ScopeData11
  Step Add (min) : Constant
  Subsystem : Subsystem
  TEST : Scope  NumInputPorts=4
      settings: ActiveDisplayYMinimum=13.625  ActiveDisplayYMaximum=27.375  DataLoggingVariableName=ScopeData3
  TEST2 : Scope  NumInputPorts=2
      settings: ActiveDisplayYMinimum=-311929.86683332996  ActiveDisplayYMaximum=2.8073688014999703E+6  DataLoggingVariableName=ScopeData4
  TMP (psi) : Sum  Inputs=|-+
  Time Since Last Backwash (min) : Integrator  ExternalReset=level hold  InitialConditionSource=external  InitialCondition=26
  Time Since Last CEB (min) : Integrator  ExternalReset=level hold  InitialConditionSource=external  InitialCondition=4833
  Time Since Last CIP (min) : Integrator  InitialCondition=round(CIP_Max_Time*rand())
  Time in Operation (only while running) : Product
  UF6_BWCompleteSignal : simulink/Logic and Bit Operations/Compare To Constant  relop===  const=1  OutDataTypeStr=uint8
  UF6_BWCycles_InitCondition : Step  Before=round(500 * rand())  After=0  SampleTime=0
  UF6_BWQualification : Logic  IconShape=distinctive  AllPortsSameDT=off  OutDataTypeStr=boolean
  UF6_BWTime_InitCondition : Step  Before=round(BW_Max_Time*rand())  After=0  SampleTime=0
  UF6_BWVol_InitCondition : Step  Before=round(BW_Max_Vol_gal*rand())  After=0  SampleTime=0
  UF6_CEBCompleteSignal : simulink/Logic and Bit Operations/Compare To Constant  relop===  const=2  OutDataTypeStr=uint8
  UF6_CEBQualification : Logic  IconShape=distinctive  AllPortsSameDT=off  OutDataTypeStr=boolean
  UF6_CEBTime_InitCondition : Step  Before=round(CEB_Max_Time*rand())  After=0  SampleTime=0
  UF6_CEBVol_InitCondition : Step  Before=round(CEB_Max_Vol_gal*rand())  After=0  SampleTime=0
  Volume Since Last Backwash (gal) : Integrator  ExternalReset=level hold  InitialConditionSource=external  InitialCondition=34330
  Volume Since Last CEB (gal) : Integrator  ExternalReset=rising  InitialConditionSource=external  InitialCondition=2777254
  "gpd -> gpm/psi" : Gain  Gain=1/1440
  Filtrate Flow (gpm) : Outport
  tag scope: UF6_Maintenance_Request=global, UF6_PermeatePressure_psi=global, UF6_gpm_psi=global
  wires:
  Volume Since Last Backwash (gal)/1 -> Subsystem/4(V_BW), TEST2/1  "V_BW"
  Time Since Last Backwash (min)/1 -> BW Maintenance Request Signal/1, Subsystem/1(t_BW), TEST/1
  Product/1 -> "gpd -> gpm/psi"/1  "UF Spec. Flow (gpd/psi)"
  [UF_MembraneCharacteristics] -> Product/2  "Membrane Area (ft^2)"
  "gpd -> gpm/psi"/1 -> Filtrate Flow Rate/1, [UF6_gpm_psi]  "Water Permeability (gpm/psi)"
  Time in Operation (only while running)/1 -> Time Since Last Backwash (min)/1, Time Since Last CEB (min)/1, Time Since Last CIP (min)/1
  Filtrate Flow Rate/1 -> Scope/1, Minus/2, Volume Since Last Backwash (gal)/1, Volume Since Last CEB (gal)/1, Compare To Constant/1, Filtrate Flow (gpm)/1  "UF6 Filtrate Flow (gpm)"
  Time Since Last CEB (min)/1 -> Subsystem/2(t_CEB), TEST/2  "t_CEB"
  Volume Since Last CEB (gal)/1 -> Subsystem/5(V_CEB), TEST2/2  "V_CEB"
  Time Since Last CIP (min)/1 -> Subsystem/3(t_CIP), TEST/3  "t_CIP"
  Filtrate Pressure MAX (psi)/1 -> Ramping Permeate Pressure/1
  [UF_Influent_WQ] -> Bus Selector/1
  Bus Selector/1 -> Subsystem/7(T)  "<UF_FeedTemperature_degC>"
  UF6_FeedFlow_Pressure/1 -> Bus Selector3/1
  Filtrate Pressure Ratio (dmnl)/1 -> Product1/1
  Product1/1 -> Ramping Permeate Pressure/2
  Ramping Permeate Pressure/1 -> [UF6_PermeatePressure_psi], TMP (psi)/1
  TMP (psi)/1 -> Filtrate Flow Rate/2
  BW Maintenance Setpoint (min)/1 -> BW Maintenance Request Signal/2
  BW Cycles Since Last CEB/1 -> GreaterThanOrEqual/1
  BW Cycles Setpoint/1 -> GreaterThanOrEqual/2
  Bus Selector/2 -> Subsystem/6(Feed Turbidity)  "<UF_FeedTurbidity_NTU>"
  [UF6_State] -> Bus Selector1/1
  MergeSignals/1 -> [UF6_Maintenance_Request]  "UF6_MaintenanceRequest"
  UF6_CEBCompleteSignal/1 -> Data Type Conversion1/1  "CEBCompleteSignal"
  [CEBCompleteSignal] -> Volume Since Last CEB (gal)/2, Time Since Last CEB (min)/2
  Data Type Conversion/1 -> [BWCompleteSignal], BW Cycles Since Last CEB/1  "BWCompleteSignal"
  [BWCompleteSignal] -> Volume Since Last Backwash (gal)/2, Time Since Last Backwash (min)/2
  [CEBCompleteSignal] -> BW Cycles Since Last CEB/2
  Bus Selector1/1 -> Memory/1  "<UF6_MaintenanceCompletion_signal>"
  UF6_BWCompleteSignal/1 -> Data Type Conversion/1  "BWCompleteSignal"
  Data Type Conversion1/1 -> [CEBCompleteSignal]  "CEBCompleteSignal"
  UF6_BWCycles_InitCondition/1 -> BW Cycles Since Last CEB/3
  Subsystem/1(A_UF) -> TEST/4, Product/1  "membrane permeability (GFD/psi)"
  UF6_BWTime_InitCondition/1 -> Time Since Last Backwash (min)/3  "T_BWInitCondition"
  UF6_CEBVol_InitCondition/1 -> Volume Since Last CEB (gal)/3
  UF6_CEBTime_InitCondition/1 -> Time Since Last CEB (min)/3
  UF6_BWVol_InitCondition/1 -> Volume Since Last Backwash (gal)/3  "V_BWInitCondition"
  Step Add (min)/1 -> Time in Operation (only while running)/1
  Compare To Constant/1 -> Time in Operation (only while running)/2
  Memory/1 -> UF6_BWCompleteSignal/1, UF6_CEBCompleteSignal/1
  UF6_BWQualification/1 -> MergeSignals/1  "UF6_BWRequest"
  GreaterThanOrEqual/1 -> UF6_CEBQualification/2  "UF6 CEB Request Signal"
  UF6_CEBQualification/1 -> CEBSignal_Level/1, NOT/1  "UF6_CEBRequest"
  BW Maintenance Request Signal/1 -> UF6_BWQualification/1, UF6_CEBQualification/1  "UF6 BW Request Signal"
  NOT/1 -> UF6_BWQualification/2
  CEBSignal_Level/1 -> MergeSignals/2  "UF6_CEBRequest"
  Bus Selector3/1 -> Scope1/2, Minus/1, Scope/3  "<UF6_FeedFlow>"
  Bus Selector3/2 -> TMP (psi)/2, Scope1/1, Product1/2  "<UF_FeedPressure_psi>"
  Minus/1 -> Scope/2  "WasteFlow_UF6"
